simulink subsystem "GeometricModel"  (R2020b)
settings: Solver=VariableStepAuto  StartTime=0.0  StopTime=10.0  RelTol=1e-3
settings Model: Creator=Master  LastModifiedBy=Master

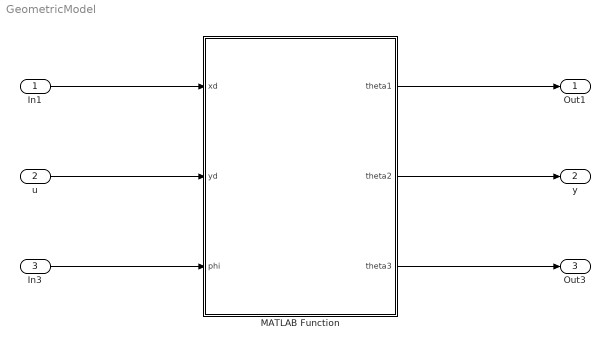
== system GeometricModel ==
  In1 : Inport
  u : Inport  Port=2
  In3 : Inport  Port=3
  MATLAB Function : MATLAB Function  TreatAsAtomicUnit=on
  Out1 : Outport
  y : Outport  Port=2
  Out3 : Outport  Port=3
  wires:
  u/1 -> MATLAB Function/2(yd)
  In1/1 -> MATLAB Function/1(xd)
  In3/1 -> MATLAB Function/3(phi)
  MATLAB Function/2(theta2) -> y/1
  MATLAB Function/1(theta1) -> Out1/1
  MATLAB Function/3(theta3) -> Out3/1

== matlab function GeometricModel/MATLAB Function ==
  data: theta1 output; xd input; yd input; theta2 output; phi input; theta3 output
function [theta1,theta2,theta3] = GeometricCalculation(xd, yd, phi)

y = yd;
